simulink model "control_pos_6dof_sinMI"  (R2023b)
settings: Solver=ode45  StartTime=0.0  StopTime=tsim  FixedStep=tstep  MaxStep=tstep  RelTol=tstep/10
undefined symbols (not defined in the file): a0, a1, robot_params, t_qeq_init, t_tr_init, tau_L, tr_ref
(part 6 of 7)

== matlab function control_pos_6dof_sinMI/Dinámica inversa (referencia)/Modelo dinámico ==
  data: robot_params input; robot_din output Bus: robot_din_bus size=1; q input size=[6,1]; dq input size=[6,1]
function robot_din = fcn(robot_params,q,dq)


% l1 = robot_params.l(1);
l2 = robot_params.l(2);
l3 = robot_params.l(3);
% l4 = robot_params.l(4);
% l5 = robot_params.l(5);
% l6 = robot_params.l(6);

lc1 = robot_params.lc(1);
lc2 = robot_params.lc(2);
lc3 = robot_params.lc(3);
% lc4 = robot_params.lc(4);
% lc5 = robot_params.lc(5);
% lc6 = robot_params.lc(6);

d1 = robot_params.d(1);
d2 = robot_params.d(2);
d3 = robot_params.d(3);
d4 = robot_params.d(4);
d5 = robot_params.d(5);
d6 = robot_params.d(6);

% dc1 = robot_params.dc(1);
% dc2 = robot_params.dc(2);
% dc3 = robot_params.dc(3);
dc4 = robot_params.dc(4);
dc5 = robot_params.dc(5);
dc6 = robot_params.dc(6);

m1 = robot_params.m(1);
m2 = robot_params.m(2);
m3 = robot_params.m(3);
m4 = robot_params.m(4);
m5 = robot_params.m(5);
m6 = robot_params.m(6);

%Posiciones angulares
% q1 = q(1);
q2 = q(2);
q3 = q(3);
q4 = q(4);
q5 = q(5);
% q6 = q(6);

%Velocidades angulares
dq1 = dq(1);
dq2 = dq(2);
dq3 = dq(3);
dq4 = dq(4);
dq5 = dq(5);
% dq6 = dq(6);

% Matriz de Inercia D
D = zeros(6,6);

D(1,1) = (d1*m1)/2 + (d2*m2)/2 + (d3*m3)/2 + (d4*m4)/2 + (d5*m5)/2 + (d6*m6)/2 + d4^2*m5 + d4^2*m6 + (d5^2*m6)/2 + dc4^2*m4 + (dc5^2*m5)/2 + (3*dc6^2*m6)/4 + (l2^2*m3)/2 + (l2^2*m4)/2 + (l2^2*m5)/2 + (l3^2*m4)/2 + (l2^2*m6)/2 + (l3^2*m5)/2 + (l3^2*m6)/2 + lc1^2*m1 + (lc2^2*m2)/2 + (lc3^2*m3)/2 - (dc6^2*m6*cos(2*q2 + 2*q3 + 2*q4 - 2*q5))/8 - (dc6^2*m6*cos(2*q2 + 2*q3 + 2*q4 + 2*q5))/8 - (d5^2*m6*cos(2*q2 + 2*q3 + 2*q4))/2 + (dc6^2*m6*cos(2*q5))/4 - (dc5^2*m5*cos(2*q2 + 2*q3 + 2*q4))/2 + (dc6^2*m6*cos(2*q2 + 2*q3 + 2*q4))/4 + (l2^2*m3*cos(2*q2))/2 + (l2^2*m4*cos(2*q2))/2 + (l2^2*m5*cos(2*q2))/2 + (l2^2*m6*cos(2*q2))/2 + (lc2^2*m2*cos(2*q2))/2 + (l3^2*m4*cos(2*q2 + 2*q3))/2 + (l3^2*m5*cos(2*q2 + 2*q3))/2 + (l3^2*m6*cos(2*q2 + 2*q3))/2 + (lc3^2*m3*cos(2*q2 + 2*q3))/2 + d5*l2*m6*sin(2*q2 + q3 + q4) + dc5*l2*m5*sin(2*q2 + q3 + q4) + (dc6*l2*m6*sin(q3 + q4 - q5))/2 + (d5*dc6*m6*cos(2*q2 + 2*q3 + 2*q4 + q5))/2 + d5*l2*m6*sin(q3 + q4) + dc5*l2*m5*sin(q3 + q4) - (dc6*l3*m6*sin(q4 + q5))/2 + (dc6*l3*m6*sin(2*q2 + 2*q3 + q4 - q5))/2 + 2*d4*dc6*m6*cos(q5) + l2*l3*m4*cos(q3) + l2*l3*m5*cos(q3) + l2*l3*m6*cos(q3) + l2*lc3*m3*cos(q3) + d5*l3*m6*sin(q4) + d5*l3*m6*sin(2*q2 + 2*q3 + q4) + dc5*l3*m5*sin(q4) + dc5*l3*m5*sin(2*q2 + 2*q3 + q4) - (dc6*l2*m6*sin(2*q2 + q3 + q4 + q5))/2 - (d5*dc6*m6*cos(2*q2 + 2*q3 + 2*q4 - q5))/2 + l2*l3*m4*cos(2*q2 + q3) + l2*l3*m5*cos(2*q2 + q3) + l2*l3*m6*cos(2*q2 + q3) + l2*lc3*m3*cos(2*q2 + q3) + (dc6*l3*m6*sin(q4 - q5))/2 - (dc6*l2*m6*sin(q3 + q4 + q5))/2 + (dc6*l2*m6*sin(2*q2 + q3 + q4 - q5))/2 - (dc6*l3*m6*sin(2*q2 + 2*q3 + q4 + q5))/2;
D(1,2) = (dc6^2*m6*cos(q2 + q3 + q4 - 2*q5))/4 - (dc6^2*m6*cos(q2 + q3 + q4 + 2*q5))/4 - (d4*dc6*m6*cos(q2 + q3 + q4 + q5))/2 + (d5*dc6*m6*cos(q2 + q3 + q4 + q5))/2 - (dc6*l3*m6*sin(q2 + q3 - q5))/2 - d4*l3*m5*sin(q2 + q3) - d4*l3*m6*sin(q2 + q3) - dc4*l3*m4*sin(q2 + q3) - (dc6*l2*m6*sin(q2 + q5))/2 + (d4*dc6*m6*cos(q2 + q3 + q4 - q5))/2 + (d5*dc6*m6*cos(q2 + q3 + q4 - q5))/2 - d4*l2*m5*sin(q2) - d4*l2*m6*sin(q2) - dc4*l2*m4*sin(q2) + d4*d5*m6*cos(q2 + q3 + q4) + d4*dc5*m5*cos(q2 + q3 + q4) - (dc6*l2*m6*sin(q2 - q5))/2 - (dc6*l3*m6*sin(q2 + q3 + q5))/2;
D(1,3) = (dc6^2*m6*cos(q2 + q3 + q4 - 2*q5))/4 - (dc6^2*m6*cos(q2 + q3 + q4 + 2*q5))/4 - (d4*dc6*m6*cos(q2 + q3 + q4 + q5))/2 + (d5*dc6*m6*cos(q2 + q3 + q4 + q5))/2 - (dc6*l3*m6*sin(q2 + q3 - q5))/2 - d4*l3*m5*sin(q2 + q3) - d4*l3*m6*sin(q2 + q3) - dc4*l3*m4*sin(q2 + q3) + (d4*dc6*m6*cos(q2 + q3 + q4 - q5))/2 + (d5*dc6*m6*cos(q2 + q3 + q4 - q5))/2 + d4*d5*m6*cos(q2 + q3 + q4) + d4*dc5*m5*cos(q2 + q3 + q4) - (dc6*l3*m6*sin(q2 + q3 + q5))/2;
D(1,4) = (dc6^2*m6*cos(q2 + q3 + q4 - 2*q5))/4 - (dc6^2*m6*cos(q2 + q3 + q4 + 2*q5))/4 - (d4*dc6*m6*cos(q2 + q3 + q4 + q5))/2 + (d5*dc6*m6*cos(q2 + q3 + q4 + q5))/2 + (d4*dc6*m6*cos(q2 + q3 + q4 - q5))/2 + (d5*dc6*m6*cos(q2 + q3 + q4 - q5))/2 + d4*d5*m6*cos(q2 + q3 + q4) + d4*dc5*m5*cos(q2 + q3 + q4);
D(1,5) = -(dc6*m6*(d4*cos(q2 + q3 + q4 + q5) + d5*cos(q2 + q3 + q4 + q5) + l3*sin(q2 + q3 - q5) - l2*sin(q2 + q5) + d4*cos(q2 + q3 + q4 - q5) - d5*cos(q2 + q3 + q4 - q5) + 2*dc6*cos(q2 + q3 + q4) + l2*sin(q2 - q5) - l3*sin(q2 + q3 + q5)))/2;
D(1,6) = 0;

D(2,1) = (dc6^2*m6*cos(q2 + q3 + q4 - 2*q5))/4 - (dc6^2*m6*cos(q2 + q3 + q4 + 2*q5))/4 - (d4*dc6*m6*cos(q2 + q3 + q4 + q5))/2 + (d5*dc6*m6*cos(q2 + q3 + q4 + q5))/2 - (dc6*l3*m6*sin(q2 + q3 - q5))/2 - d4*l3*m5*sin(q2 + q3) - d4*l3*m6*sin(q2 + q3) - dc4*l3*m4*sin(q2 + q3) - (dc6*l2*m6*sin(q2 + q5))/2 + (d4*dc6*m6*cos(q2 + q3 + q4 - q5))/2 + (d5*dc6*m6*cos(q2 + q3 + q4 - q5))/2 - d4*l2*m5*sin(q2) - d4*l2*m6*sin(q2) - dc4*l2*m4*sin(q2) + d4*d5*m6*cos(q2 + q3 + q4) + d4*dc5*m5*cos(q2 + q3 + q4) - (dc6*l2*m6*sin(q2 - q5))/2 - (dc6*l3*m6*sin(q2 + q3 + q5))/2;
D(2,2) = (d2*m2)/2 + (d3*m3)/2 + (d4*m4)/2 + (d5*m5)/2 + (d6*m6)/2 + d5^2*m6 + dc5^2*m5 + (dc6^2*m6)/2 + l2^2*m3 + l2^2*m4 + l2^2*m5 + l3^2*m4 + l2^2*m6 + l3^2*m5 + l3^2*m6 + lc2^2*m2 + lc3^2*m3 - (dc6^2*m6*cos(2*q5))/2 + 2*d5*l2*m6*sin(q3 + q4) + 2*dc5*l2*m5*sin(q3 + q4) + 2*l2*l3*m4*cos(q3) + 2*l2*l3*m5*cos(q3) + 2*l2*l3*m6*cos(q3) + 2*l2*lc3*m3*cos(q3) + 2*d5*l3*m6*sin(q4) + 2*dc5*l3*m5*sin(q4) - 2*dc6*l3*m6*cos(q4)*sin(q5) - 2*dc6*l2*m6*cos(q3)*cos(q4)*sin(q5) + 2*dc6*l2*m6*sin(q3)*sin(q4)*sin(q5);
D(2,3) = d5^2*m6 + dc5^2*m5 + (dc6^2*m6)/2 + l3^2*m4 + l3^2*m5 + l3^2*m6 + lc3^2*m3 - (dc6^2*m6*cos(2*q5))/2 + d5*l2*m6*sin(q3 + q4) + dc5*l2*m5*sin(q3 + q4) + l2*l3*m4*cos(q3) + l2*l3*m5*cos(q3) + l2*l3*m6*cos(q3) + l2*lc3*m3*cos(q3) + 2*d5*l3*m6*sin(q4) + 2*dc5*l3*m5*sin(q4) - 2*dc6*l3*m6*cos(q4)*sin(q5) - dc6*l2*m6*cos(q3)*cos(q4)*sin(q5) + dc6*l2*m6*sin(q3)*sin(q4)*sin(q5);
D(2,4) = d5^2*m6 + dc5^2*m5 + (dc6^2*m6)/2 - (dc6^2*m6*cos(2*q5))/2 + d5*l2*m6*sin(q3 + q4) + dc5*l2*m5*sin(q3 + q4) + d5*l3*m6*sin(q4) + dc5*l3*m5*sin(q4) - dc6*l3*m6*cos(q4)*sin(q5) - dc6*l2*m6*cos(q3)*cos(q4)*sin(q5) + dc6*l2*m6*sin(q3)*sin(q4)*sin(q5);
D(2,5) = -dc6*m6*cos(q5)*(d5 + l2*sin(q3 + q4) + l3*sin(q4));
D(2,6) = 0;

D(3,1) = (dc6^2*m6*cos(q2 + q3 + q4 - 2*q5))/4 - (dc6^2*m6*cos(q2 + q3 + q4 + 2*q5))/4 - (d4*dc6*m6*cos(q2 + q3 + q4 + q5))/2 + (d5*dc6*m6*cos(q2 + q3 + q4 + q5))/2 - (dc6*l3*m6*sin(q2 + q3 - q5))/2 - d4*l3*m5*sin(q2 + q3) - d4*l3*m6*sin(q2 + q3) - dc4*l3*m4*sin(q2 + q3) + (d4*dc6*m6*cos(q2 + q3 + q4 - q5))/2 + (d5*dc6*m6*cos(q2 + q3 + q4 - q5))/2 + d4*d5*m6*cos(q2 + q3 + q4) + d4*dc5*m5*cos(q2 + q3 + q4) - (dc6*l3*m6*sin(q2 + q3 + q5))/2;
D(3,2) = d5^2*m6 + dc5^2*m5 + (dc6^2*m6)/2 + l3^2*m4 + l3^2*m5 + l3^2*m6 + lc3^2*m3 - (dc6^2*m6*cos(2*q5))/2 + d5*l2*m6*sin(q3 + q4) + dc5*l2*m5*sin(q3 + q4) + l2*l3*m4*cos(q3) + l2*l3*m5*cos(q3) + l2*l3*m6*cos(q3) + l2*lc3*m3*cos(q3) + 2*d5*l3*m6*sin(q4) + 2*dc5*l3*m5*sin(q4) - 2*dc6*l3*m6*cos(q4)*sin(q5) - dc6*l2*m6*cos(q3)*cos(q4)*sin(q5) + dc6*l2*m6*sin(q3)*sin(q4)*sin(q5);
D(3,3) = (d3*m3)/2 + (d4*m4)/2 + (d5*m5)/2 + (d6*m6)/2 + d5^2*m6 + dc5^2*m5 + l3^2*m4 + l3^2*m5 + l3^2*m6 + lc3^2*m3 + dc6^2*m6*sin(q5)^2 + 2*d5*l3*m6*sin(q4) + 2*dc5*l3*m5*sin(q4) - 2*dc6*l3*m6*cos(q4)*sin(q5);
D(3,4) = d5^2*m6 + dc5^2*m5 + dc6^2*m6*sin(q5)^2 + d5*l3*m6*sin(q4) + dc5*l3*m5*sin(q4) - dc6*l3*m6*cos(q4)*sin(q5);
D(3,5) = -dc6*m6*cos(q5)*(d5 + l3*sin(q4));
D(3,6) = 0;

D(4,1) = (dc6^2*m6*cos(q2 + q3 + q4 - 2*q5))/4 - (dc6^2*m6*cos(q2 + q3 + q4 + 2*q5))/4 - (d4*dc6*m6*cos(q2 + q3 + q4 + q5))/2 + (d5*dc6*m6*cos(q2 + q3 + q4 + q5))/2 + (d4*dc6*m6*cos(q2 + q3 + q4 - q5))/2 + (d5*dc6*m6*cos(q2 + q3 + q4 - q5))/2 + d4*d5*m6*cos(q2 + q3 + q4) + d4*dc5*m5*cos(q2 + q3 + q4);
D(4,2) = d5^2*m6 + dc5^2*m5 + (dc6^2*m6)/2 - (dc6^2*m6*cos(2*q5))/2 + d5*l2*m6*sin(q3 + q4) + dc5*l2*m5*sin(q3 + q4) + d5*l3*m6*sin(q4) + dc5*l3*m5*sin(q4) - dc6*l3*m6*cos(q4)*sin(q5) - dc6*l2*m6*cos(q3)*cos(q4)*sin(q5) + dc6*l2*m6*sin(q3)*sin(q4)*sin(q5);
D(4,3) = d5^2*m6 + dc5^2*m5 + dc6^2*m6*sin(q5)^2 + d5*l3*m6*sin(q4) + dc5*l3*m5*sin(q4) - dc6*l3*m6*cos(q4)*sin(q5);
D(4,4) = (d4*m4)/2 + (d5*m5)/2 + (d6*m6)/2 + d5^2*m6 + dc5^2*m5 + dc6^2*m6 - dc6^2*m6*cos(q5)^2;
D(4,5) = -d5*dc6*m6*cos(q5);
D(4,6) = 0;

D(5,1) = -(dc6*m6*(d4*cos(q2 + q3 + q4 + q5) + d5*cos(q2 + q3 + q4 + q5) + l3*sin(q2 + q3 - q5) - l2*sin(q2 + q5) + d4*cos(q2 + q3 + q4 - q5) - d5*cos(q2 + q3 + q4 - q5) + 2*dc6*cos(q2 + q3 + q4) + l2*sin(q2 - q5) - l3*sin(q2 + q3 + q5)))/2;
D(5,2) = -dc6*m6*cos(q5)*(d5 + l2*sin(q3 + q4) + l3*sin(q4));
D(5,3) = -dc6*m6*cos(q5)*(d5 + l3*sin(q4));
D(5,4) = -d5*dc6*m6*cos(q5);
D(5,5) = (d5*m5)/2 + (d6*m6)/2 + dc6^2*m6;
D(5,6) = 0;

D(6,1) = 0;
D(6,2) = 0;
D(6,3) = 0;
D(6,4) = 0;
D(6,5) = 0;
D(6,6) = 1;


% Matriz de Coriollis C
C = zeros(6,6);

C(1,1) = 0;
C(1,2) = (dc6^2*dq1*m6*sin(2*q2 + 2*q3 + 2*q4 - 2*q5))/4 + (dc6^2*dq1*m6*sin(2*q2 + 2*q3 + 2*q4 + 2*q5))/4 + d5^2*dq1*m6*sin(2*q2 + 2*q3 + 2*q4) + dc5^2*dq1*m5*sin(2*q2 + 2*q3 + 2*q4) - (dc6^2*dq1*m6*sin(2*q2 + 2*q3 + 2*q4))/2 - dq1*l2^2*m3*sin(2*q2) - dq1*l2^2*m4*sin(2*q2) - dq1*l2^2*m5*sin(2*q2) - dq1*l2^2*m6*sin(2*q2) - dq1*lc2^2*m2*sin(2*q2) - dq1*l3^2*m4*sin(2*q2 + 2*q3) - dq1*l3^2*m5*sin(2*q2 + 2*q3) - dq1*l3^2*m6*sin(2*q2 + 2*q3) - dq1*lc3^2*m3*sin(2*q2 + 2*q3) - (dc6^2*dq2*m6*sin(q2 + q3 + q4 - 2*q5))/4 + (dc6^2*dq2*m6*sin(q2 + q3 + q4 + 2*q5))/4 - (dc6*dq2*l2*m6*cos(q2 - q5))/2 + d5*dc6*dq1*m6*sin(2*q2 + 2*q3 + 2*q4 - q5) - (dc6*dq2*l3*m6*cos(q2 + q3 + q5))/2 - 2*dq1*l2*l3*m4*sin(2*q2 + q3) - 2*dq1*l2*l3*m5*sin(2*q2 + q3) - 2*dq1*l2*l3*m6*sin(2*q2 + q3) - 2*dq1*l2*lc3*m3*sin(2*q2 + q3) - d4*d5*dq2*m6*sin(q2 + q3 + q4) - d4*dc5*dq2*m5*sin(q2 + q3 + q4) + dc6*dq1*l2*m6*cos(2*q2 + q3 + q4 - q5) - dc6*dq1*l3*m6*cos(2*q2 + 2*q3 + q4 + q5) + 2*d5*dq1*l2*m6*cos(2*q2 + q3 + q4) + 2*dc5*dq1*l2*m5*cos(2*q2 + q3 + q4) - (dc6*dq2*l3*m6*cos(q2 + q3 - q5))/2 + (d4*dc6*dq2*m6*sin(q2 + q3 + q4 + q5))/2 - (d5*dc6*dq2*m6*sin(q2 + q3 + q4 + q5))/2 - d4*dq2*l3*m5*cos(q2 + q3) - d4*dq2*l3*m6*cos(q2 + q3) - dc4*dq2*l3*m4*cos(q2 + q3) - (dc6*dq2*l2*m6*cos(q2 + q5))/2 + dc6*dq1*l3*m6*cos(2*q2 + 2*q3 + q4 - q5) - d5*dc6*dq1*m6*sin(2*q2 + 2*q3 + 2*q4 + q5) - d4*dq2*l2*m5*cos(q2) - d4*dq2*l2*m6*cos(q2) + 2*d5*dq1*l3*m6*cos(2*q2 + 2*q3 + q4) - dc4*dq2*l2*m4*cos(q2) + 2*dc5*dq1*l3*m5*cos(2*q2 + 2*q3 + q4) - dc6*dq1*l2*m6*cos(2*q2 + q3 + q4 + q5) - (d4*dc6*dq2*m6*sin(q2 + q3 + q4 - q5))/2 - (d5*dc6*dq2*m6*sin(q2 + q3 + q4 - q5))/2;
C(1,3) = (dc6^2*dq1*m6*sin(2*q2 + 2*q3 + 2*q4 - 2*q5))/4 + (dc6^2*dq1*m6*sin(2*q2 + 2*q3 + 2*q4 + 2*q5))/4 + d5^2*dq1*m6*sin(2*q2 + 2*q3 + 2*q4) + dc5^2*dq1*m5*sin(2*q2 + 2*q3 + 2*q4) - (dc6^2*dq1*m6*sin(2*q2 + 2*q3 + 2*q4))/2 - dq1*l3^2*m4*sin(2*q2 + 2*q3) - dq1*l3^2*m5*sin(2*q2 + 2*q3) - dq1*l3^2*m6*sin(2*q2 + 2*q3) - dq1*lc3^2*m3*sin(2*q2 + 2*q3) - (dc6^2*dq2*m6*sin(q2 + q3 + q4 - 2*q5))/2 + (dc6^2*dq2*m6*sin(q2 + q3 + q4 + 2*q5))/2 - (dc6^2*dq3*m6*sin(q2 + q3 + q4 - 2*q5))/4 + (dc6^2*dq3*m6*sin(q2 + q3 + q4 + 2*q5))/4 + d5*dc6*dq1*m6*sin(2*q2 + 2*q3 + 2*q4 - q5) - (dc6*dq1*l2*m6*cos(q3 + q4 + q5))/2 - dc6*dq2*l3*m6*cos(q2 + q3 + q5) - (dc6*dq3*l3*m6*cos(q2 + q3 + q5))/2 - dq1*l2*l3*m4*sin(2*q2 + q3) - dq1*l2*l3*m5*sin(2*q2 + q3) - dq1*l2*l3*m6*sin(2*q2 + q3) - dq1*l2*lc3*m3*sin(2*q2 + q3) - 2*d4*d5*dq2*m6*sin(q2 + q3 + q4) - d4*d5*dq3*m6*sin(q2 + q3 + q4) - 2*d4*dc5*dq2*m5*sin(q2 + q3 + q4) - d4*dc5*dq3*m5*sin(q2 + q3 + q4) + (dc6*dq1*l2*m6*cos(2*q2 + q3 + q4 - q5))/2 - dc6*dq1*l3*m6*cos(2*q2 + 2*q3 + q4 + q5) + d5*dq1*l2*m6*cos(2*q2 + q3 + q4) + dc5*dq1*l2*m5*cos(2*q2 + q3 + q4) + (dc6*dq1*l2*m6*cos(q3 + q4 - q5))/2 - dc6*dq2*l3*m6*cos(q2 + q3 - q5) - (dc6*dq3*l3*m6*cos(q2 + q3 - q5))/2 + d4*dc6*dq2*m6*sin(q2 + q3 + q4 + q5) + (d4*dc6*dq3*m6*sin(q2 + q3 + q4 + q5))/2 - d5*dc6*dq2*m6*sin(q2 + q3 + q4 + q5) - (d5*dc6*dq3*m6*sin(q2 + q3 + q4 + q5))/2 - 2*d4*dq2*l3*m5*cos(q2 + q3) - 2*d4*dq2*l3*m6*cos(q2 + q3) - d4*dq3*l3*m5*cos(q2 + q3) - d4*dq3*l3*m6*cos(q2 + q3) + d5*dq1*l2*m6*cos(q3 + q4) - 2*dc4*dq2*l3*m4*cos(q2 + q3) - dc4*dq3*l3*m4*cos(q2 + q3) + dc5*dq1*l2*m5*cos(q3 + q4) + dc6*dq1*l3*m6*cos(2*q2 + 2*q3 + q4 - q5) - d5*dc6*dq1*m6*sin(2*q2 + 2*q3 + 2*q4 + q5) + 2*d5*dq1*l3*m6*cos(2*q2 + 2*q3 + q4) + 2*dc5*dq1*l3*m5*cos(2*q2 + 2*q3 + q4) - (dc6*dq1*l2*m6*cos(2*q2 + q3 + q4 + q5))/2 - dq1*l2*l3*m4*sin(q3) - dq1*l2*l3*m5*sin(q3) - dq1*l2*l3*m6*sin(q3) - dq1*l2*lc3*m3*sin(q3) - d4*dc6*dq2*m6*sin(q2 + q3 + q4 - q5) - (d4*dc6*dq3*m6*sin(q2 + q3 + q4 - q5))/2 - d5*dc6*dq2*m6*sin(q2 + q3 + q4 - q5) - (d5*dc6*dq3*m6*sin(q2 + q3 + q4 - q5))/2;
C(1,4) = (dc6^2*dq1*m6*sin(2*q2 + 2*q3 + 2*q4 - 2*q5))/4 + (dc6^2*dq1*m6*sin(2*q2 + 2*q3 + 2*q4 + 2*q5))/4 + d5^2*dq1*m6*sin(2*q2 + 2*q3 + 2*q4) + dc5^2*dq1*m5*sin(2*q2 + 2*q3 + 2*q4) - (dc6^2*dq1*m6*sin(2*q2 + 2*q3 + 2*q4))/2 - (dc6^2*dq2*m6*sin(q2 + q3 + q4 - 2*q5))/2 + (dc6^2*dq2*m6*sin(q2 + q3 + q4 + 2*q5))/2 - (dc6^2*dq3*m6*sin(q2 + q3 + q4 - 2*q5))/2 + (dc6^2*dq3*m6*sin(q2 + q3 + q4 + 2*q5))/2 - (dc6^2*dq4*m6*sin(q2 + q3 + q4 - 2*q5))/4 + (dc6^2*dq4*m6*sin(q2 + q3 + q4 + 2*q5))/4 + (dc6*dq1*l3*m6*cos(q4 - q5))/2 + d5*dc6*dq1*m6*sin(2*q2 + 2*q3 + 2*q4 - q5) - (dc6*dq1*l2*m6*cos(q3 + q4 + q5))/2 - 2*d4*d5*dq2*m6*sin(q2 + q3 + q4) - 2*d4*d5*dq3*m6*sin(q2 + q3 + q4) - d4*d5*dq4*m6*sin(q2 + q3 + q4) - 2*d4*dc5*dq2*m5*sin(q2 + q3 + q4) - 2*d4*dc5*dq3*m5*sin(q2 + q3 + q4) - d4*dc5*dq4*m5*sin(q2 + q3 + q4) + (dc6*dq1*l2*m6*cos(2*q2 + q3 + q4 - q5))/2 - (dc6*dq1*l3*m6*cos(2*q2 + 2*q3 + q4 + q5))/2 + d5*dq1*l2*m6*cos(2*q2 + q3 + q4) + dc5*dq1*l2*m5*cos(2*q2 + q3 + q4) + (dc6*dq1*l2*m6*cos(q3 + q4 - q5))/2 + d4*dc6*dq2*m6*sin(q2 + q3 + q4 + q5) + d4*dc6*dq3*m6*sin(q2 + q3 + q4 + q5) - d5*dc6*dq2*m6*sin(q2 + q3 + q4 + q5) + (d4*dc6*dq4*m6*sin(q2 + q3 + q4 + q5))/2 - d5*dc6*dq3*m6*sin(q2 + q3 + q4 + q5) - (d5*dc6*dq4*m6*sin(q2 + q3 + q4 + q5))/2 + d5*dq1*l2*m6*cos(q3 + q4) + dc5*dq1*l2*m5*cos(q3 + q4) - (dc6*dq1*l3*m6*cos(q4 + q5))/2 + (dc6*dq1*l3*m6*cos(2*q2 + 2*q3 + q4 - q5))/2 - d5*dc6*dq1*m6*sin(2*q2 + 2*q3 + 2*q4 + q5) + d5*dq1*l3*m6*cos(q4) + d5*dq1*l3*m6*cos(2*q2 + 2*q3 + q4) + dc5*dq1*l3*m5*cos(q4) + dc5*dq1*l3*m5*cos(2*q2 + 2*q3 + q4) - (dc6*dq1*l2*m6*cos(2*q2 + q3 + q4 + q5))/2 - d4*dc6*dq2*m6*sin(q2 + q3 + q4 - q5) - d4*dc6*dq3*m6*sin(q2 + q3 + q4 - q5) - d5*dc6*dq2*m6*sin(q2 + q3 + q4 - q5) - (d4*dc6*dq4*m6*sin(q2 + q3 + q4 - q5))/2 - d5*dc6*dq3*m6*sin(q2 + q3 + q4 - q5) - (d5*dc6*dq4*m6*sin(q2 + q3 + q4 - q5))/2;
C(1,5) = (dc6*m6*(4*d4*dq2*sin(q2 + q3 + q4 - q5) - 2*dq1*l2*cos(2*q2 + q3 + q4 + q5) - 8*d4*dq1*sin(q5) + 4*d4*dq3*sin(q2 + q3 + q4 - q5) + 4*d4*dq4*sin(q2 + q3 + q4 - q5) - 2*d4*dq5*sin(q2 + q3 + q4 - q5) + 2*d5*dq5*sin(q2 + q3 + q4 - q5) + 2*dc6*dq2*sin(q2 + q3 + q4 - 2*q5) + 2*dc6*dq2*sin(q2 + q3 + q4 + 2*q5) + 2*dc6*dq3*sin(q2 + q3 + q4 - 2*q5) + 2*dc6*dq3*sin(q2 + q3 + q4 + 2*q5) + 2*dc6*dq4*sin(q2 + q3 + q4 - 2*q5) + 2*dc6*dq4*sin(q2 + q3 + q4 + 2*q5) - 2*dq1*l3*cos(q4 - q5) + 2*dq5*l2*cos(q2 - q5) - 2*d5*dq1*sin(2*q2 + 2*q3 + 2*q4 - q5) - dc6*dq1*sin(2*q2 + 2*q3 + 2*q4 - 2*q5) + dc6*dq1*sin(2*q2 + 2*q3 + 2*q4 + 2*q5) - 2*dq1*l2*cos(q3 + q4 + q5) + 2*dq5*l3*cos(q2 + q3 + q5) + 4*dc6*dq2*sin(q2 + q3 + q4) + 4*dc6*dq3*sin(q2 + q3 + q4) + 4*dc6*dq4*sin(q2 + q3 + q4) - 2*dc6*dq1*sin(2*q5) - 2*dq1*l2*cos(2*q2 + q3 + q4 - q5) - 2*dq1*l3*cos(2*q2 + 2*q3 + q4 + q5) - 2*dq1*l2*cos(q3 + q4 - q5) + 2*dq5*l3*cos(q2 + q3 - q5) + 4*d4*dq2*sin(q2 + q3 + q4 + q5) + 4*d4*dq3*sin(q2 + q3 + q4 + q5) + 4*d4*dq4*sin(q2 + q3 + q4 + q5) + 2*d4*dq5*sin(q2 + q3 + q4 + q5) + 2*d5*dq5*sin(q2 + q3 + q4 + q5) - 2*dq1*l3*cos(q4 + q5) + 2*dq5*l2*cos(q2 + q5) - 2*dq1*l3*cos(2*q2 + 2*q3 + q4 - q5) - 2*d5*dq1*sin(2*q2 + 2*q3 + 2*q4 + q5)))/4;
C(1,6) = 0;

C(2,1) = (dc6^2*dq1*m6*sin(2*q2 + 2*q3 + 2*q4))/4 - (dc6^2*dq1*m6*sin(2*q2 + 2*q3 + 2*q4 + 2*q5))/8 - (d5^2*dq1*m6*sin(2*q2 + 2*q3 + 2*q4))/2 - (dc5^2*dq1*m5*sin(2*q2 + 2*q3 + 2*q4))/2 - (dc6^2*dq1*m6*sin(2*q2 + 2*q3 + 2*q4 - 2*q5))/8 + (dq1*l2^2*m3*sin(2*q2))/2 + (dq1*l2^2*m4*sin(2*q2))/2 + (dq1*l2^2*m5*sin(2*q2))/2 + (dq1*l2^2*m6*sin(2*q2))/2 + (dq1*lc2^2*m2*sin(2*q2))/2 + (dq1*l3^2*m4*sin(2*q2 + 2*q3))/2 + (dq1*l3^2*m5*sin(2*q2 + 2*q3))/2 + (dq1*l3^2*m6*sin(2*q2 + 2*q3))/2 + (dq1*lc3^2*m3*sin(2*q2 + 2*q3))/2 - (d5*dc6*dq1*m6*sin(2*q2 + 2*q3 + 2*q4 - q5))/2 + dq1*l2*l3*m4*sin(2*q2 + q3) + dq1*l2*l3*m5*sin(2*q2 + q3) + dq1*l2*l3*m6*sin(2*q2 + q3) + dq1*l2*lc3*m3*sin(2*q2 + q3) - (dc6*dq1*l2*m6*cos(2*q2 + q3 + q4 - q5))/2 + (dc6*dq1*l3*m6*cos(2*q2 + 2*q3 + q4 + q5))/2 - d5*dq1*l2*m6*cos(2*q2 + q3 + q4) - dc5*dq1*l2*m5*cos(2*q2 + q3 + q4) - (dc6*dq1*l3*m6*cos(2*q2 + 2*q3 + q4 - q5))/2 + (d5*dc6*dq1*m6*sin(2*q2 + 2*q3 + 2*q4 + q5))/2 - d5*dq1*l3*m6*cos(2*q2 + 2*q3 + q4) - dc5*dq1*l3*m5*cos(2*q2 + 2*q3 + q4) + (dc6*dq1*l2*m6*cos(2*q2 + q3 + q4 + q5))/2;
C(2,2) = 0;
C(2,3) = -l2*(2*dq2 + dq3)*(l3*m4*sin(q3) + l3*m5*sin(q3) + l3*m6*sin(q3) + lc3*m3*sin(q3) - d5*m6*cos(q3 + q4) - dc5*m5*cos(q3 + q4) - dc6*m6*cos(q3)*sin(q4)*sin(q5) - dc6*m6*cos(q4)*sin(q3)*sin(q5));
C(2,4) = (dc6*dq4*l3*m6*cos(q4 - q5))/2 + 2*d5*dq2*l2*m6*cos(q3 + q4) + 2*d5*dq3*l2*m6*cos(q3 + q4) + d5*dq4*l2*m6*cos(q3 + q4) + 2*dc5*dq2*l2*m5*cos(q3 + q4) + 2*dc5*dq3*l2*m5*cos(q3 + q4) + dc5*dq4*l2*m5*cos(q3 + q4) - (dc6*dq4*l3*m6*cos(q4 + q5))/2 + 2*d5*dq2*l3*m6*cos(q4) + 2*d5*dq3*l3*m6*cos(q4) + d5*dq4*l3*m6*cos(q4) + 2*dc5*dq2*l3*m5*cos(q4) + 2*dc5*dq3*l3*m5*cos(q4) + dc5*dq4*l3*m5*cos(q4) + 2*dc6*dq2*l3*m6*sin(q4)*sin(q5) + 2*dc6*dq3*l3*m6*sin(q4)*sin(q5) + 2*dc6*dq2*l2*m6*cos(q3)*sin(q4)*sin(q5) + 2*dc6*dq2*l2*m6*cos(q4)*sin(q3)*sin(q5) + 2*dc6*dq3*l2*m6*cos(q3)*sin(q4)*sin(q5) + 2*dc6*dq3*l2*m6*cos(q4)*sin(q3)*sin(q5) + dc6*dq4*l2*m6*cos(q3)*sin(q4)*sin(q5) + dc6*dq4*l2*m6*cos(q4)*sin(q3)*sin(q5);
C(2,5) = -(dc6*m6*(2*dq2*l3*cos(q4 - q5) - 2*d5*dq1*sin(q2 + q3 + q4 - q5) - dc6*dq1*sin(q2 + q3 + q4 - 2*q5) - dc6*dq1*sin(q2 + q3 + q4 + 2*q5) - 2*dq1*l2*cos(q2 - q5) - 2*d5*dq5*sin(q5) + 2*dq3*l3*cos(q4 - q5) + 2*dq4*l3*cos(q4 - q5) - dq5*l3*cos(q4 - q5) + 2*dq1*l3*cos(q2 + q3 + q5) + 2*dq2*l2*cos(q3 + q4 + q5) + 2*dq3*l2*cos(q3 + q4 + q5) + 2*dq4*l2*cos(q3 + q4 + q5) + dq5*l2*cos(q3 + q4 + q5) + 2*dc6*dq1*sin(q2 + q3 + q4) - 2*dc6*dq2*sin(2*q5) - 2*dc6*dq3*sin(2*q5) - 2*dc6*dq4*sin(2*q5) - 2*dq1*l3*cos(q2 + q3 - q5) + 2*dq2*l2*cos(q3 + q4 - q5) + 2*dq3*l2*cos(q3 + q4 - q5) + 2*dq4*l2*cos(q3 + q4 - q5) - dq5*l2*cos(q3 + q4 - q5) + 2*d5*dq1*sin(q2 + q3 + q4 + q5) + 2*dq1*l2*cos(q2 + q5) + 2*dq2*l3*cos(q4 + q5) + 2*dq3*l3*cos(q4 + q5) + 2*dq4*l3*cos(q4 + q5) + dq5*l3*cos(q4 + q5)))/2;
C(2,6) = 0;

C(3,1) = (dc6^2*dq1*m6*sin(2*q2 + 2*q3 + 2*q4))/4 - (dc6^2*dq1*m6*sin(2*q2 + 2*q3 + 2*q4 + 2*q5))/8 - (d5^2*dq1*m6*sin(2*q2 + 2*q3 + 2*q4))/2 - (dc5^2*dq1*m5*sin(2*q2 + 2*q3 + 2*q4))/2 - (dc6^2*dq1*m6*sin(2*q2 + 2*q3 + 2*q4 - 2*q5))/8 + (dq1*l3^2*m4*sin(2*q2 + 2*q3))/2 + (dq1*l3^2*m5*sin(2*q2 + 2*q3))/2 + (dq1*l3^2*m6*sin(2*q2 + 2*q3))/2 + (dq1*lc3^2*m3*sin(2*q2 + 2*q3))/2 - (d5*dc6*dq1*m6*sin(2*q2 + 2*q3 + 2*q4 - q5))/2 + (dc6*dq1*l2*m6*cos(q3 + q4 + q5))/4 + (dq1*l2*l3*m4*sin(2*q2 + q3))/2 + (dq1*l2*l3*m5*sin(2*q2 + q3))/2 + (dq1*l2*l3*m6*sin(2*q2 + q3))/2 + (dq1*l2*lc3*m3*sin(2*q2 + q3))/2 - (dc6*dq1*l2*m6*cos(2*q2 + q3 + q4 - q5))/4 + (dc6*dq1*l3*m6*cos(2*q2 + 2*q3 + q4 + q5))/2 - (d5*dq1*l2*m6*cos(2*q2 + q3 + q4))/2 - (dc5*dq1*l2*m5*cos(2*q2 + q3 + q4))/2 - (dc6*dq1*l2*m6*cos(q3 + q4 - q5))/4 - (d5*dq1*l2*m6*cos(q3 + q4))/2 - (dc5*dq1*l2*m5*cos(q3 + q4))/2 - (dc6*dq1*l3*m6*cos(2*q2 + 2*q3 + q4 - q5))/2 + (d5*dc6*dq1*m6*sin(2*q2 + 2*q3 + 2*q4 + q5))/2 - d5*dq1*l3*m6*cos(2*q2 + 2*q3 + q4) - dc5*dq1*l3*m5*cos(2*q2 + 2*q3 + q4) + (dc6*dq1*l2*m6*cos(2*q2 + q3 + q4 + q5))/4 + (dq1*l2*l3*m4*sin(q3))/2 + (dq1*l2*l3*m5*sin(q3))/2 + (dq1*l2*l3*m6*sin(q3))/2 + (dq1*l2*lc3*m3*sin(q3))/2;
C(3,2) = dq2*l2*(l3*m4*sin(q3) + l3*m5*sin(q3) + l3*m6*sin(q3) + lc3*m3*sin(q3) - d5*m6*cos(q3 + q4) - dc5*m5*cos(q3 + q4) - dc6*m6*cos(q3)*sin(q4)*sin(q5) - dc6*m6*cos(q4)*sin(q3)*sin(q5));
C(3,3) = 0;
C(3,4) = l3*(2*dq2 + 2*dq3 + dq4)*(d5*m6*cos(q4) + dc5*m5*cos(q4) + dc6*m6*sin(q4)*sin(q5));
C(3,5) = -dc6*m6*(dq2*l3*cos(q4 - q5) - d5*dq1*sin(q2 + q3 + q4 - q5) - (dc6*dq1*sin(q2 + q3 + q4 - 2*q5))/2 - (dc6*dq1*sin(q2 + q3 + q4 + 2*q5))/2 - d5*dq5*sin(q5) + dq3*l3*cos(q4 - q5) + dq4*l3*cos(q4 - q5) - (dq5*l3*cos(q4 - q5))/2 + dq1*l3*cos(q2 + q3 + q5) + dc6*dq1*sin(q2 + q3 + q4) - dc6*dq2*sin(2*q5) - dc6*dq3*sin(2*q5) - dc6*dq4*sin(2*q5) - dq1*l3*cos(q2 + q3 - q5) + d5*dq1*sin(q2 + q3 + q4 + q5) + dq2*l3*cos(q4 + q5) + dq3*l3*cos(q4 + q5) + dq4*l3*cos(q4 + q5) + (dq5*l3*cos(q4 + q5))/2);
C(3,6) = 0;

C(4,1) = (dc6^2*dq1*m6*sin(2*q2 + 2*q3 + 2*q4))/4 - (dc6^2*dq1*m6*sin(2*q2 + 2*q3 + 2*q4 + 2*q5))/8 - (d5^2*dq1*m6*sin(2*q2 + 2*q3 + 2*q4))/2 - (dc5^2*dq1*m5*sin(2*q2 + 2*q3 + 2*q4))/2 - (dc6^2*dq1*m6*sin(2*q2 + 2*q3 + 2*q4 - 2*q5))/8 - (dc6*dq1*l3*m6*cos(q4 - q5))/4 - (d5*dc6*dq1*m6*sin(2*q2 + 2*q3 + 2*q4 - q5))/2 + (dc6*dq1*l2*m6*cos(q3 + q4 + q5))/4 - (dc6*dq1*l2*m6*cos(2*q2 + q3 + q4 - q5))/4 + (dc6*dq1*l3*m6*cos(2*q2 + 2*q3 + q4 + q5))/4 - (d5*dq1*l2*m6*cos(2*q2 + q3 + q4))/2 - (dc5*dq1*l2*m5*cos(2*q2 + q3 + q4))/2 - (dc6*dq1*l2*m6*cos(q3 + q4 - q5))/4 - (d5*dq1*l2*m6*cos(q3 + q4))/2 - (dc5*dq1*l2*m5*cos(q3 + q4))/2 + (dc6*dq1*l3*m6*cos(q4 + q5))/4 - (dc6*dq1*l3*m6*cos(2*q2 + 2*q3 + q4 - q5))/4 + (d5*dc6*dq1*m6*sin(2*q2 + 2*q3 + 2*q4 + q5))/2 - (d5*dq1*l3*m6*cos(q4))/2 - (d5*dq1*l3*m6*cos(2*q2 + 2*q3 + q4))/2 - (dc5*dq1*l3*m5*cos(q4))/2 - (dc5*dq1*l3*m5*cos(2*q2 + 2*q3 + q4))/2 + (dc6*dq1*l2*m6*cos(2*q2 + q3 + q4 + q5))/4;
C(4,2) = - dq2*(l2*cos(q3 + q4) + l3*cos(q4))*(d5*m6 + dc5*m5) - dc6*dq2*l3*m6*sin(q4)*sin(q5) - dc6*dq2*l2*m6*cos(q3)*sin(q4)*sin(q5) - dc6*dq2*l2*m6*cos(q4)*sin(q3)*sin(q5);
C(4,3) = -l3*(2*dq2 + dq3)*(d5*m6*cos(q4) + dc5*m5*cos(q4) + dc6*m6*sin(q4)*sin(q5));
C(4,4) = 0;
C(4,5) = (dc6*m6*(2*d5*dq5*sin(q5) + 2*d5*dq1*sin(q2 + q3 + q4 - q5) + dc6*dq1*sin(q2 + q3 + q4 - 2*q5) + dc6*dq1*sin(q2 + q3 + q4 + 2*q5) - 2*dc6*dq1*sin(q2 + q3 + q4) + 2*dc6*dq2*sin(2*q5) + 2*dc6*dq3*sin(2*q5) + 2*dc6*dq4*sin(2*q5) - 2*d5*dq1*sin(q2 + q3 + q4 + q5)))/2;
C(4,6) = 0;

C(5,1) = (dc6*dq1*m6*(2*dc6*sin(2*q5) + 2*l2*cos(2*q2 + q3 + q4 - q5) + 2*l3*cos(2*q2 + 2*q3 + q4 + q5) + 2*l2*cos(q3 + q4 - q5) + 2*l3*cos(q4 + q5) + 2*l3*cos(2*q2 + 2*q3 + q4 - q5) + 2*d5*sin(2*q2 + 2*q3 + 2*q4 + q5) + 8*d4*sin(q5) + 2*l2*cos(2*q2 + q3 + q4 + q5) + 2*l3*cos(q4 - q5) + 2*d5*sin(2*q2 + 2*q3 + 2*q4 - q5) + dc6*sin(2*q2 + 2*q3 + 2*q4 - 2*q5) - dc6*sin(2*q2 + 2*q3 + 2*q4 + 2*q5) + 2*l2*cos(q3 + q4 + q5)))/8;
C(5,2) = (dc6*m6*(dq2*l3*cos(q4 - q5) - dc6*dq1*sin(q2 + q3 + q4 - 2*q5) - dc6*dq1*sin(q2 + q3 + q4 + 2*q5) - 2*dq1*l2*cos(q2 - q5) - 2*d5*dq1*sin(q2 + q3 + q4 - q5) + 2*dq1*l3*cos(q2 + q3 + q5) + dq2*l2*cos(q3 + q4 + q5) + 2*dc6*dq1*sin(q2 + q3 + q4) - dc6*dq2*sin(2*q5) - 2*dq1*l3*cos(q2 + q3 - q5) + dq2*l2*cos(q3 + q4 - q5) + 2*d5*dq1*sin(q2 + q3 + q4 + q5) + 2*dq1*l2*cos(q2 + q5) + dq2*l3*cos(q4 + q5)))/2;
C(5,3) = (dc6*m6*(2*dq2*l3*cos(q4 - q5) - dc6*dq1*sin(q2 + q3 + q4 - 2*q5) - dc6*dq1*sin(q2 + q3 + q4 + 2*q5) - 2*d5*dq1*sin(q2 + q3 + q4 - q5) + dq3*l3*cos(q4 - q5) + 2*dq1*l3*cos(q2 + q3 + q5) + 2*dc6*dq1*sin(q2 + q3 + q4) - 2*dc6*dq2*sin(2*q5) - dc6*dq3*sin(2*q5) - 2*dq1*l3*cos(q2 + q3 - q5) + 2*d5*dq1*sin(q2 + q3 + q4 + q5) + 2*dq2*l3*cos(q4 + q5) + dq3*l3*cos(q4 + q5)))/2;
C(5,4) = -(dc6*m6*(2*d5*dq1*sin(q2 + q3 + q4 - q5) + dc6*dq1*sin(q2 + q3 + q4 - 2*q5) + dc6*dq1*sin(q2 + q3 + q4 + 2*q5) - 2*dc6*dq1*sin(q2 + q3 + q4) + 2*dc6*dq2*sin(2*q5) + 2*dc6*dq3*sin(2*q5) + dc6*dq4*sin(2*q5) - 2*d5*dq1*sin(q2 + q3 + q4 + q5)))/2;
C(5,5) = 0;
C(5,6) = 0;

C(6,1) = 0;
C(6,2) = 0;
C(6,3) = 0;
C(6,4) = 0;
C(6,5) = 0;
C(6,6) = 0;


% Matriz de Gravedad G: 
G = zeros(6,1);

G(1,1) = 0;

G(2,1) = l2*m3*cos(q2) + l2*m4*cos(q2) + l2*m5*cos(q2) + l2*m6*cos(q2) + lc2*m2*cos(q2) + (dc6*m6*sin(q2 + q3 + q4 - q5))/2 + d5*m6*sin(q2 + q3 + q4) + dc5*m5*sin(q2 + q3 + q4) - (dc6*m6*sin(q2 + q3 + q4 + q5))/2 + l3*m4*cos(q2 + q3) + l3*m5*cos(q2 + q3) + l3*m6*cos(q2 + q3) + lc3*m3*cos(q2 + q3);

G(3,1) = (dc6*m6*sin(q2 + q3 + q4 - q5))/2 + d5*m6*sin(q2 + q3 + q4) + dc5*m5*sin(q2 + q3 + q4) - (dc6*m6*sin(q2 + q3 + q4 + q5))/2 + l3*m4*cos(q2 + q3) + l3*m5*cos(q2 + q3) + l3*m6*cos(q2 + q3) + lc3*m3*cos(q2 + q3);

G(4,1) = (dc6*m6*sin(q2 + q3 + q4 - q5))/2 + d5*m6*sin(q2 + q3 + q4) + dc5*m5*sin(q2 + q3 + q4) - (dc6*m6*sin(q2 + q3 + q4 + q5))/2;

G(5,1) = -(dc6*m6*(sin(q2 + q3 + q4 + q5) + sin(q2 + q3 + q4 - q5)))/2;

G(6,1) = 0;

robot_din = struct('D',D,'C',C,'G',G,'g',9.81);

%busInfo = Simulink.Bus.createObject(robot_dyn);

== matlab function control_pos_6dof_sinMI/q to xyz (referencia)/Cinemática directa ==
  data: robot_params input; p output; q input
function p = fcn(robot_params,q)

l1 = robot_params.l(1);
l2 = robot_params.l(2);
l3 = robot_params.l(3);
l4 = robot_params.l(4);
l5 = robot_params.l(5);
l6 = robot_params.l(6);

d1 = robot_params.d(1);
d2 = robot_params.d(2);
d3 = robot_params.d(3);
d4 = robot_params.d(4);
d5 = robot_params.d(5);
d6 = robot_params.d(6);

q1 = q(1);
q2 = q(2);
q3 = q(3);
q4 = q(4);
q5 = q(5);
q6 = q(6);

% Cinematica directa %%%%%%%%%%%%%%%%%%%%%%%%%%%%%%%%%%%%%%%%%%%%%%%%%%%%%%

DH = [0   pi/2  d1 q1;
      l2  0     0  q2;
      l3  0     0  q3;
      0   pi/2  d4 q4;
      0   -pi/2 d5 q5;
      0   0     d6 q6];

A01 = transformacion_homogenea(DH(1,:));
A12 = transformacion_homogenea(DH(2,:));
A23 = transformacion_homogenea(DH(3,:));
A34 = transformacion_homogenea(DH(4,:));
A45 = transformacion_homogenea(DH(5,:));
A56 = transformacion_homogenea(DH(6,:));

T0 = zeros(4,4,6);

T0(:,:,1) = A01;
T0(:,:,2) = A01*A12;
T0(:,:,3) = A01*A12*A23;
T0(:,:,4) = A01*A12*A23*A34;
T0(:,:,5) = A01*A12*A23*A34*A45;
T0(:,:,6) = A01*A12*A23*A34*A45*A56;

p = reshape(T0(1:3,4,:),[3,6]);

end

function m = transformacion_homogenea(DH_i)
    a_i = DH_i(1);
    alpha_i = DH_i(2);
    d_i = DH_i(3);
    theta_i = DH_i(4);
    
    ma_i = [1 0 0 a_i;
            0 1 0 0;
            0 0 1 0;
            0 0 0 1];
    
    md_i = [1 0 0 0;
            0 1 0 0;
            0 0 1 d_i;
            0 0 0 1];
    
    mtheta_i = [cos(theta_i) -sin(theta_i) 0 0;
                sin(theta_i) cos(theta_i) 0 0;
                0 0 1 0;
                0 0 0 1];
    
    malpha_i = [1 0 0 0;
                0 cos(alpha_i) -sin(alpha_i) 0;
                0 sin(alpha_i) cos(alpha_i) 0;
                0 0 0 1];
    
    m = mtheta_i * md_i * ma_i * malpha_i;

end

== matlab function control_pos_6dof_sinMI/q to xyz (referencia)/Jacobiano ==
  data: robot_params input; q input; JP output
function JP = JP(robot_params,q)

%l1 = robot_params.l(1);
l2 = robot_params.l(2);
l3 = robot_params.l(3);
%l4 = robot_params.l(4);
%l5 = robot_params.l(5);
%l6 = robot_params.l(6);

lc1 = robot_params.lc(1);
lc2 = robot_params.lc(2);
lc3 = robot_params.lc(3);
%lc4 = robot_params.lc(4);
%lc5 = robot_params.lc(5);
%lc6 = robot_params.lc(6);

d1 = robot_params.d(1);
%d2 = robot_params.d(2);
%d3 = robot_params.d(3);
d4 = robot_params.d(4);
d5 = robot_params.d(5);
%d6 = robot_params.d(6);

dc1 = robot_params.dc(1);
%dc2 = robot_params.dc(2);
%dc3 = robot_params.dc(3);
dc4 = robot_params.dc(4);
dc5 = robot_params.dc(5);
dc6 = robot_params.dc(6);

q1 = q(1);
q2 = q(2);
q3 = q(3);
q4 = q(4);
q5 = q(5);
%q6 = q(6);

% Cinematica diferencial %%%%%%%%%%%%%%%%%%%%%%%%%%%%%%%%%%%%%%%%%%%%%%%%%%

JP = zeros(3,6);

JP(1,1) = -cos(q1)*(d1 + l3*sin(q2 + q3) + l2*sin(q2) - d5*cos(q2 + q3 + q4) - dc6*sin(q2 + q3 + q4)*sin(q5));
JP(1,2) = -cos(q1)*(d1 - dc1 + l3*sin(q2 + q3) + l2*sin(q2) - d5*cos(q2 + q3 + q4) - dc6*sin(q2 + q3 + q4)*sin(q5));
JP(1,3) = cos(q1)*(lc2*sin(q2) - l2*sin(q2) - l3*sin(q2 + q3) + d5*cos(q2 + q3 + q4) + dc6*sin(q2 + q3 + q4)*sin(q5));
JP(1,4) = - cos(q2 + q3 + q4)*(dc6*(cos(q1)*cos(q5) + cos(q2 + q3 + q4)*sin(q1)*sin(q5)) + d4*cos(q1) - sin(q1)*(l3*cos(q2 + q3) + l2*cos(q2)) + sin(q1)*(lc3*cos(q2 + q3) + l2*cos(q2)) - d5*sin(q2 + q3 + q4)*sin(q1)) - sin(q2 + q3 + q4)*sin(q1)*(lc3*sin(q2 + q3) - l3*sin(q2 + q3) + d5*cos(q2 + q3 + q4) + dc6*sin(q2 + q3 + q4)*sin(q5));
JP(1,5) = d5*sin(q1)*sin(q5) + d5*cos(q2 + q3 + q4)*cos(q1)*cos(q5) - d4*sin(q2 + q3 + q4)*cos(q1)*sin(q5) + dc4*sin(q2 + q3 + q4)*cos(q1)*sin(q5);
JP(1,6) = (d5 - dc5)*(sin(q1)*sin(q5) + cos(q2 + q3 + q4)*cos(q1)*cos(q5));

JP(2,1) = -sin(q1)*(d1 + l3*sin(q2 + q3) + l2*sin(q2) - d5*cos(q2 + q3 + q4) - dc6*sin(q2 + q3 + q4)*sin(q5));
JP(2,2) = -sin(q1)*(d1 - dc1 + l3*sin(q2 + q3) + l2*sin(q2) - d5*cos(q2 + q3 + q4) - dc6*sin(q2 + q3 + q4)*sin(q5));
JP(2,3) = sin(q1)*(lc2*sin(q2) - l2*sin(q2) - l3*sin(q2 + q3) + d5*cos(q2 + q3 + q4) + dc6*sin(q2 + q3 + q4)*sin(q5));
JP(2,4) = sin(q2 + q3 + q4)*cos(q1)*(lc3*sin(q2 + q3) - l3*sin(q2 + q3) + d5*cos(q2 + q3 + q4) + dc6*sin(q2 + q3 + q4)*sin(q5)) - cos(q2 + q3 + q4)*(dc6*(cos(q5)*sin(q1) - cos(q2 + q3 + q4)*cos(q1)*sin(q5)) + cos(q1)*(l3*cos(q2 + q3) + l2*cos(q2)) - cos(q1)*(lc3*cos(q2 + q3) + l2*cos(q2)) + d4*sin(q1) + d5*sin(q2 + q3 + q4)*cos(q1));
JP(2,5) = d5*cos(q2 + q3 + q4)*cos(q5)*sin(q1) - d5*cos(q1)*sin(q5) - d4*sin(q2 + q3 + q4)*sin(q1)*sin(q5) + dc4*sin(q2 + q3 + q4)*sin(q1)*sin(q5);
JP(2,6) = -(d5 - dc5)*(cos(q1)*sin(q5) - cos(q2 + q3 + q4)*cos(q5)*sin(q1));

JP(3,1) = l3*cos(q2 + q3) - (dc6*sin(q2 + q3 + q4 + q5))/2 + l2*cos(q2) + (dc6*sin(q2 + q3 + q4 - q5))/2 + d5*sin(q2 + q3 + q4);
JP(3,2) = l3*cos(q2 + q3) - (dc6*sin(q2 + q3 + q4 + q5))/2 - lc1 + l2*cos(q2) + (dc6*sin(q2 + q3 + q4 - q5))/2 + d5*sin(q2 + q3 + q4);
JP(3,3) = l3*cos(q2 + q3) - (dc6*sin(q2 + q3 + q4 + q5))/2 + l2*cos(q2) - lc2*cos(q2) + (dc6*sin(q2 + q3 + q4 - q5))/2 + d5*sin(q2 + q3 + q4);
JP(3,4) = - (dc6*sin(q2 + q3 + q4 + q5))/2 - (dc6*sin(q2 + q3 + q4 - q5))/2 - d4*sin(q2 + q3 + q4);
JP(3,5) = d4*cos(q2 + q3 + q4)*sin(q5) + d5*sin(q2 + q3 + q4)*cos(q5) - dc4*cos(q2 + q3 + q4)*sin(q5);
JP(3,6) = sin(q2 + q3 + q4)*cos(q5)*(d5 - dc5);

== matlab function control_pos_6dof_sinMI/q to xyz (referencia)/ddq to ddp ==
  data: dJP input; ddp output; ddq input
function ddp = fcn(dJP,ddq)

ddp = dJP*ddq;

== matlab function control_pos_6dof_sinMI/q to xyz (referencia)/derivada Jacobiano ==
  data: robot_params input; q input; dJP output; dq input
function dJP = dJP(robot_params,q,dq)

%l1 = robot_params.l(1);
l2 = robot_params.l(2);
l3 = robot_params.l(3);
%l4 = robot_params.l(4);
%l5 = robot_params.l(5);
%l6 = robot_params.l(6);

lc1 = robot_params.lc(1);
lc2 = robot_params.lc(2);
lc3 = robot_params.lc(3);
%lc4 = robot_params.lc(4);
%lc5 = robot_params.lc(5);
%lc6 = robot_params.lc(6);

d1 = robot_params.d(1);
%d2 = robot_params.d(2);
%d3 = robot_params.d(3);
d4 = robot_params.d(4);
d5 = robot_params.d(5);
%d6 = robot_params.d(6);

dc1 = robot_params.dc(1);
%dc2 = robot_params.dc(2);
%dc3 = robot_params.dc(3);
dc4 = robot_params.dc(4);
dc5 = robot_params.dc(5);
dc6 = robot_params.dc(6);

dq1 = dq(1);
dq2 = dq(2);
dq3 = dq(3);
dq4 = dq(4);
dq5 = dq(5);
%dq6 = dq(6);

q1 = q(1);
q2 = q(2);
q3 = q(3);
q4 = q(4);
q5 = q(5);
%q6 = q(6);

dJP = zeros(3,6);

dJP(1,1) = dq1*sin(q1)*(d1 + l3*sin(q2 + q3) + l2*sin(q2) - d5*cos(q2 + q3 + q4) - dc6*sin(q2 + q3 + q4)*sin(q5)) - dq3*cos(q1)*(l3*cos(q2 + q3) + d5*sin(q2 + q3 + q4) - dc6*cos(q2 + q3 + q4)*sin(q5)) - dq4*cos(q1)*(d5*sin(q2 + q3 + q4) - dc6*cos(q2 + q3 + q4)*sin(q5)) - dq2*cos(q1)*(l3*cos(q2 + q3) + l2*cos(q2) + d5*sin(q2 + q3 + q4) - dc6*cos(q2 + q3 + q4)*sin(q5)) + dc6*dq5*sin(q2 + q3 + q4)*cos(q1)*cos(q5);
dJP(1,2) = dq1*sin(q1)*(d1 - dc1 + l3*sin(q2 + q3) + l2*sin(q2) - d5*cos(q2 + q3 + q4) - dc6*sin(q2 + q3 + q4)*sin(q5)) - dq3*cos(q1)*(l3*cos(q2 + q3) + d5*sin(q2 + q3 + q4) - dc6*cos(q2 + q3 + q4)*sin(q5)) - dq4*cos(q1)*(d5*sin(q2 + q3 + q4) - dc6*cos(q2 + q3 + q4)*sin(q5)) - dq2*cos(q1)*(l3*cos(q2 + q3) + l2*cos(q2) + d5*sin(q2 + q3 + q4) - dc6*cos(q2 + q3 + q4)*sin(q5)) + dc6*dq5*sin(q2 + q3 + q4)*cos(q1)*cos(q5);
dJP(1,3) = dc6*dq5*sin(q2 + q3 + q4)*cos(q1)*cos(q5) - dq2*cos(q1)*(l3*cos(q2 + q3) + l2*cos(q2) - lc2*cos(q2) + d5*sin(q2 + q3 + q4) - dc6*cos(q2 + q3 + q4)*sin(q5)) - dq1*sin(q1)*(lc2*sin(q2) - l2*sin(q2) - l3*sin(q2 + q3) + d5*cos(q2 + q3 + q4) + dc6*sin(q2 + q3 + q4)*sin(q5)) - dq4*cos(q1)*(d5*sin(q2 + q3 + q4) - dc6*cos(q2 + q3 + q4)*sin(q5)) - dq3*cos(q1)*(l3*cos(q2 + q3) + d5*sin(q2 + q3 + q4) - dc6*cos(q2 + q3 + q4)*sin(q5));
dJP(1,4) = dq1*l3*cos(q1)*cos(q4) - dq1*lc3*cos(q1)*cos(q4) - dc6*dq1*cos(q1)*sin(q5) - dc6*dq5*cos(q5)*sin(q1) - dq4*l3*sin(q1)*sin(q4) + dq4*lc3*sin(q1)*sin(q4) + d4*dq1*cos(q2)*cos(q3)*cos(q4)*sin(q1) + d4*dq2*cos(q1)*cos(q2)*cos(q3)*sin(q4) + d4*dq2*cos(q1)*cos(q2)*cos(q4)*sin(q3) + d4*dq2*cos(q1)*cos(q3)*cos(q4)*sin(q2) + d4*dq3*cos(q1)*cos(q2)*cos(q3)*sin(q4) + d4*dq3*cos(q1)*cos(q2)*cos(q4)*sin(q3) + d4*dq3*cos(q1)*cos(q3)*cos(q4)*sin(q2) + d4*dq4*cos(q1)*cos(q2)*cos(q3)*sin(q4) + d4*dq4*cos(q1)*cos(q2)*cos(q4)*sin(q3) + d4*dq4*cos(q1)*cos(q3)*cos(q4)*sin(q2) - d4*dq1*cos(q2)*sin(q1)*sin(q3)*sin(q4) - d4*dq1*cos(q3)*sin(q1)*sin(q2)*sin(q4) - d4*dq1*cos(q4)*sin(q1)*sin(q2)*sin(q3) - d4*dq2*cos(q1)*sin(q2)*sin(q3)*sin(q4) - d4*dq3*cos(q1)*sin(q2)*sin(q3)*sin(q4) - d4*dq4*cos(q1)*sin(q2)*sin(q3)*sin(q4) + dc6*dq1*cos(q2)*cos(q3)*cos(q4)*cos(q5)*sin(q1) + dc6*dq2*cos(q1)*cos(q2)*cos(q3)*cos(q5)*sin(q4) + dc6*dq2*cos(q1)*cos(q2)*cos(q4)*cos(q5)*sin(q3) + dc6*dq2*cos(q1)*cos(q3)*cos(q4)*cos(q5)*sin(q2) + dc6*dq3*cos(q1)*cos(q2)*cos(q3)*cos(q5)*sin(q4) + dc6*dq3*cos(q1)*cos(q2)*cos(q4)*cos(q5)*sin(q3) + dc6*dq3*cos(q1)*cos(q3)*cos(q4)*cos(q5)*sin(q2) + dc6*dq4*cos(q1)*cos(q2)*cos(q3)*cos(q5)*sin(q4) + dc6*dq4*cos(q1)*cos(q2)*cos(q4)*cos(q5)*sin(q3) + dc6*dq4*cos(q1)*cos(q3)*cos(q4)*cos(q5)*sin(q2) + dc6*dq5*cos(q1)*cos(q2)*cos(q3)*cos(q4)*sin(q5) - dc6*dq1*cos(q2)*cos(q5)*sin(q1)*sin(q3)*sin(q4) - dc6*dq1*cos(q3)*cos(q5)*sin(q1)*sin(q2)*sin(q4) - dc6*dq1*cos(q4)*cos(q5)*sin(q1)*sin(q2)*sin(q3) - dc6*dq2*cos(q1)*cos(q5)*sin(q2)*sin(q3)*sin(q4) - dc6*dq3*cos(q1)*cos(q5)*sin(q2)*sin(q3)*sin(q4) - dc6*dq4*cos(q1)*cos(q5)*sin(q2)*sin(q3)*sin(q4) - dc6*dq5*cos(q1)*cos(q2)*sin(q3)*sin(q4)*sin(q5) - dc6*dq5*cos(q1)*cos(q3)*sin(q2)*sin(q4)*sin(q5) - dc6*dq5*cos(q1)*cos(q4)*sin(q2)*sin(q3)*sin(q5);
dJP(1,5) = dq5*(d5*cos(q5)*sin(q1) - d4*sin(q2 + q3 + q4)*cos(q1)*cos(q5) - d5*cos(q2 + q3 + q4)*cos(q1)*sin(q5) + dc4*sin(q2 + q3 + q4)*cos(q1)*cos(q5)) + dq1*(d5*cos(q1)*sin(q5) - d5*cos(q2 + q3 + q4)*cos(q5)*sin(q1) + d4*sin(q2 + q3 + q4)*sin(q1)*sin(q5) - dc4*sin(q2 + q3 + q4)*sin(q1)*sin(q5)) - dq2*cos(q1)*(d4*cos(q2 + q3 + q4)*sin(q5) + d5*sin(q2 + q3 + q4)*cos(q5) - dc4*cos(q2 + q3 + q4)*sin(q5)) - dq3*cos(q1)*(d4*cos(q2 + q3 + q4)*sin(q5) + d5*sin(q2 + q3 + q4)*cos(q5) - dc4*cos(q2 + q3 + q4)*sin(q5)) - dq4*cos(q1)*(d4*cos(q2 + q3 + q4)*sin(q5) + d5*sin(q2 + q3 + q4)*cos(q5) - dc4*cos(q2 + q3 + q4)*sin(q5));
dJP(1,6) = dq1*(d5 - dc5)*(cos(q1)*sin(q5) - cos(q2 + q3 + q4)*cos(q5)*sin(q1)) + dq5*(d5 - dc5)*(cos(q5)*sin(q1) - cos(q2 + q3 + q4)*cos(q1)*sin(q5)) - dq2*sin(q2 + q3 + q4)*cos(q1)*cos(q5)*(d5 - dc5) - dq3*sin(q2 + q3 + q4)*cos(q1)*cos(q5)*(d5 - dc5) - dq4*sin(q2 + q3 + q4)*cos(q1)*cos(q5)*(d5 - dc5);

dJP(2,1) = dc6*dq5*sin(q2 + q3 + q4)*cos(q5)*sin(q1) - dq1*cos(q1)*(d1 + l3*sin(q2 + q3) + l2*sin(q2) - d5*cos(q2 + q3 + q4) - dc6*sin(q2 + q3 + q4)*sin(q5)) - dq4*sin(q1)*(d5*sin(q2 + q3 + q4) - dc6*cos(q2 + q3 + q4)*sin(q5)) - dq2*sin(q1)*(l3*cos(q2 + q3) + l2*cos(q2) + d5*sin(q2 + q3 + q4) - dc6*cos(q2 + q3 + q4)*sin(q5)) - dq3*sin(q1)*(l3*cos(q2 + q3) + d5*sin(q2 + q3 + q4) - dc6*cos(q2 + q3 + q4)*sin(q5));
dJP(2,2) = dc6*dq5*sin(q2 + q3 + q4)*cos(q5)*sin(q1) - dq4*sin(q1)*(d5*sin(q2 + q3 + q4) - dc6*cos(q2 + q3 + q4)*sin(q5)) - dq2*sin(q1)*(l3*cos(q2 + q3) + l2*cos(q2) + d5*sin(q2 + q3 + q4) - dc6*cos(q2 + q3 + q4)*sin(q5)) - dq1*cos(q1)*(d1 - dc1 + l3*sin(q2 + q3) + l2*sin(q2) - d5*cos(q2 + q3 + q4) - dc6*sin(q2 + q3 + q4)*sin(q5)) - dq3*sin(q1)*(l3*cos(q2 + q3) + d5*sin(q2 + q3 + q4) - dc6*cos(q2 + q3 + q4)*sin(q5));
dJP(2,3) = dq1*cos(q1)*(lc2*sin(q2) - l2*sin(q2) - l3*sin(q2 + q3) + d5*cos(q2 + q3 + q4) + dc6*sin(q2 + q3 + q4)*sin(q5)) - dq2*sin(q1)*(l3*cos(q2 + q3) + l2*cos(q2) - lc2*cos(q2) + d5*sin(q2 + q3 + q4) - dc6*cos(q2 + q3 + q4)*sin(q5)) - dq3*sin(q1)*(l3*cos(q2 + q3) + d5*sin(q2 + q3 + q4) - dc6*cos(q2 + q3 + q4)*sin(q5)) - dq4*sin(q1)*(d5*sin(q2 + q3 + q4) - dc6*cos(q2 + q3 + q4)*sin(q5)) + dc6*dq5*sin(q2 + q3 + q4)*cos(q5)*sin(q1);
dJP(2,4) = dc6*dq5*cos(q1)*cos(q5) + dq1*l3*cos(q4)*sin(q1) + dq4*l3*cos(q1)*sin(q4) - dq1*lc3*cos(q4)*sin(q1) - dq4*lc3*cos(q1)*sin(q4) - dc6*dq1*sin(q1)*sin(q5) - d4*dq1*cos(q1)*cos(q2)*cos(q3)*cos(q4) + d4*dq1*cos(q1)*cos(q2)*sin(q3)*sin(q4) + d4*dq1*cos(q1)*cos(q3)*sin(q2)*sin(q4) + d4*dq1*cos(q1)*cos(q4)*sin(q2)*sin(q3) + d4*dq2*cos(q2)*cos(q3)*sin(q1)*sin(q4) + d4*dq2*cos(q2)*cos(q4)*sin(q1)*sin(q3) + d4*dq2*cos(q3)*cos(q4)*sin(q1)*sin(q2) + d4*dq3*cos(q2)*cos(q3)*sin(q1)*sin(q4) + d4*dq3*cos(q2)*cos(q4)*sin(q1)*sin(q3) + d4*dq3*cos(q3)*cos(q4)*sin(q1)*sin(q2) + d4*dq4*cos(q2)*cos(q3)*sin(q1)*sin(q4) + d4*dq4*cos(q2)*cos(q4)*sin(q1)*sin(q3) + d4*dq4*cos(q3)*cos(q4)*sin(q1)*sin(q2) - d4*dq2*sin(q1)*sin(q2)*sin(q3)*sin(q4) - d4*dq3*sin(q1)*sin(q2)*sin(q3)*sin(q4) - d4*dq4*sin(q1)*sin(q2)*sin(q3)*sin(q4) - dc6*dq1*cos(q1)*cos(q2)*cos(q3)*cos(q4)*cos(q5) + dc6*dq1*cos(q1)*cos(q2)*cos(q5)*sin(q3)*sin(q4) + dc6*dq1*cos(q1)*cos(q3)*cos(q5)*sin(q2)*sin(q4) + dc6*dq1*cos(q1)*cos(q4)*cos(q5)*sin(q2)*sin(q3) + dc6*dq2*cos(q2)*cos(q3)*cos(q5)*sin(q1)*sin(q4) + dc6*dq2*cos(q2)*cos(q4)*cos(q5)*sin(q1)*sin(q3) + dc6*dq2*cos(q3)*cos(q4)*cos(q5)*sin(q1)*sin(q2) + dc6*dq3*cos(q2)*cos(q3)*cos(q5)*sin(q1)*sin(q4) + dc6*dq3*cos(q2)*cos(q4)*cos(q5)*sin(q1)*sin(q3) + dc6*dq3*cos(q3)*cos(q4)*cos(q5)*sin(q1)*sin(q2) + dc6*dq4*cos(q2)*cos(q3)*cos(q5)*sin(q1)*sin(q4) + dc6*dq4*cos(q2)*cos(q4)*cos(q5)*sin(q1)*sin(q3) + dc6*dq4*cos(q3)*cos(q4)*cos(q5)*sin(q1)*sin(q2) + dc6*dq5*cos(q2)*cos(q3)*cos(q4)*sin(q1)*sin(q5) - dc6*dq2*cos(q5)*sin(q1)*sin(q2)*sin(q3)*sin(q4) - dc6*dq3*cos(q5)*sin(q1)*sin(q2)*sin(q3)*sin(q4) - dc6*dq4*cos(q5)*sin(q1)*sin(q2)*sin(q3)*sin(q4) - dc6*dq5*cos(q2)*sin(q1)*sin(q3)*sin(q4)*sin(q5) - dc6*dq5*cos(q3)*sin(q1)*sin(q2)*sin(q4)*sin(q5) - dc6*dq5*cos(q4)*sin(q1)*sin(q2)*sin(q3)*sin(q5);
dJP(2,5) = dq1*(d5*sin(q1)*sin(q5) + d5*cos(q2 + q3 + q4)*cos(q1)*cos(q5) - d4*sin(q2 + q3 + q4)*cos(q1)*sin(q5) + dc4*sin(q2 + q3 + q4)*cos(q1)*sin(q5)) - dq5*(d5*cos(q1)*cos(q5) + d4*sin(q2 + q3 + q4)*cos(q5)*sin(q1) + d5*cos(q2 + q3 + q4)*sin(q1)*sin(q5) - dc4*sin(q2 + q3 + q4)*cos(q5)*sin(q1)) - dq2*sin(q1)*(d4*cos(q2 + q3 + q4)*sin(q5) + d5*sin(q2 + q3 + q4)*cos(q5) - dc4*cos(q2 + q3 + q4)*sin(q5)) - dq3*sin(q1)*(d4*cos(q2 + q3 + q4)*sin(q5) + d5*sin(q2 + q3 + q4)*cos(q5) - dc4*cos(q2 + q3 + q4)*sin(q5)) - dq4*sin(q1)*(d4*cos(q2 + q3 + q4)*sin(q5) + d5*sin(q2 + q3 + q4)*cos(q5) - dc4*cos(q2 + q3 + q4)*sin(q5));
dJP(2,6) = dq1*(d5 - dc5)*(sin(q1)*sin(q5) + cos(q2 + q3 + q4)*cos(q1)*cos(q5)) - dq5*(d5 - dc5)*(cos(q1)*cos(q5) + cos(q2 + q3 + q4)*sin(q1)*sin(q5)) - dq2*sin(q2 + q3 + q4)*cos(q5)*sin(q1)*(d5 - dc5) - dq3*sin(q2 + q3 + q4)*cos(q5)*sin(q1)*(d5 - dc5) - dq4*sin(q2 + q3 + q4)*cos(q5)*sin(q1)*(d5 - dc5);

dJP(3,1) = dq4*((dc6*cos(q2 + q3 + q4 - q5))/2 - (dc6*cos(q2 + q3 + q4 + q5))/2 + d5*cos(q2 + q3 + q4)) - dq3*((dc6*cos(q2 + q3 + q4 + q5))/2 + l3*sin(q2 + q3) - (dc6*cos(q2 + q3 + q4 - q5))/2 - d5*cos(q2 + q3 + q4)) - dq2*((dc6*cos(q2 + q3 + q4 + q5))/2 + l3*sin(q2 + q3) - (dc6*cos(q2 + q3 + q4 - q5))/2 + l2*sin(q2) - d5*cos(q2 + q3 + q4)) - (dc6*dq5*(cos(q2 + q3 + q4 + q5) + cos(q2 + q3 + q4 - q5)))/2;
dJP(3,2) = dq4*((dc6*cos(q2 + q3 + q4 - q5))/2 - (dc6*cos(q2 + q3 + q4 + q5))/2 + d5*cos(q2 + q3 + q4)) - dq3*((dc6*cos(q2 + q3 + q4 + q5))/2 + l3*sin(q2 + q3) - (dc6*cos(q2 + q3 + q4 - q5))/2 - d5*cos(q2 + q3 + q4)) - dq2*((dc6*cos(q2 + q3 + q4 + q5))/2 + l3*sin(q2 + q3) - (dc6*cos(q2 + q3 + q4 - q5))/2 + l2*sin(q2) - d5*cos(q2 + q3 + q4)) - (dc6*dq5*(cos(q2 + q3 + q4 + q5) + cos(q2 + q3 + q4 - q5)))/2;
dJP(3,3) = dq4*((dc6*cos(q2 + q3 + q4 - q5))/2 - (dc6*cos(q2 + q3 + q4 + q5))/2 + d5*cos(q2 + q3 + q4)) - dq3*((dc6*cos(q2 + q3 + q4 + q5))/2 + l3*sin(q2 + q3) - (dc6*cos(q2 + q3 + q4 - q5))/2 - d5*cos(q2 + q3 + q4)) - dq2*((dc6*cos(q2 + q3 + q4 + q5))/2 + l3*sin(q2 + q3) - (dc6*cos(q2 + q3 + q4 - q5))/2 + l2*sin(q2) - lc2*sin(q2) - d5*cos(q2 + q3 + q4)) - dq5*((dc6*cos(q2 + q3 + q4 + q5))/2 + (dc6*cos(q2 + q3 + q4 - q5))/2);
dJP(3,4) = - dq2*((dc6*cos(q2 + q3 + q4 + q5))/2 + (dc6*cos(q2 + q3 + q4 - q5))/2 + d4*cos(q2 + q3 + q4)) - dq3*((dc6*cos(q2 + q3 + q4 + q5))/2 + (dc6*cos(q2 + q3 + q4 - q5))/2 + d4*cos(q2 + q3 + q4)) - dq4*((dc6*cos(q2 + q3 + q4 + q5))/2 + (dc6*cos(q2 + q3 + q4 - q5))/2 + d4*cos(q2 + q3 + q4)) - (dc6*dq5*(cos(q2 + q3 + q4 + q5) - cos(q2 + q3 + q4 - q5)))/2;
dJP(3,5) = dq2*(d5*cos(q2 + q3 + q4)*cos(q5) - d4*sin(q2 + q3 + q4)*sin(q5) + dc4*sin(q2 + q3 + q4)*sin(q5)) - dq5*(dc4*cos(q2 + q3 + q4)*cos(q5) - d4*cos(q2 + q3 + q4)*cos(q5) + d5*sin(q2 + q3 + q4)*sin(q5)) + dq3*(d5*cos(q2 + q3 + q4)*cos(q5) - d4*sin(q2 + q3 + q4)*sin(q5) + dc4*sin(q2 + q3 + q4)*sin(q5)) + dq4*(d5*cos(q2 + q3 + q4)*cos(q5) - d4*sin(q2 + q3 + q4)*sin(q5) + dc4*sin(q2 + q3 + q4)*sin(q5));
dJP(3,6) = (d5 - dc5)*(dq2*cos(q2 + q3 + q4)*cos(q5) + dq3*cos(q2 + q3 + q4)*cos(q5) + dq4*cos(q2 + q3 + q4)*cos(q5) - dq5*sin(q2 + q3 + q4)*sin(q5));

== matlab function control_pos_6dof_sinMI/q to xyz (referencia)/dq to dp ==
  data: JP input; dp output; dq input
function dp = fcn(JP,dq)

dp = JP*dq;
